simulink model "rp5p1"  (Simulink 10.1)
settings: Solver=ode5  StartTime=0.0  StopTime=10  FixedStep=0.001  RelTol=1e-3
libraries: simulink x3, Solver_SF x1
settings Model: Creator=lancer  LastModifiedBy=Administrator
settings DataIOCC: SaveFormat=Dataset
settings OptimizationCC: LifeSpan=auto
settings DebuggingCC: UnderspecifiedInitializationDetection=Simplified  MergeDetectMultiDrivingBlocksExec=error  SFUnexpectedBacktrackingDiag=error  SFNoUnconditionalDefaultTransitionDiag=error  SFExecutionAtInitializationDiag=warning
settings HardwareCC: ProdBitPerPointer=64  ProdBitPerSizeT=64  ProdBitPerPtrDiffT=64  ProdLargestAtomicFloat=Float  ProdIntDivRoundTo=Zero  ProdEndianess=LittleEndian  ProdWordSize=64  ProdHWDeviceType=Intel->x86-64 (Windows64)
settings ModelReferenceCC: PropagateSignalLabelsOutOfModel=on
settings CodeAppCC: StateflowObjectComments=off
settings GRTTargetCC: TargetLangStandard=C99 (ISO)  CombineOutputUpdateFcns=on  GRTInterface=off
settings ConfigComp: CovMetricSettings=dwe  CovHtmlReporting=off  CovSaveCumulativeToWorkspaceVar=off  CovSaveSingleToWorkspaceVar=off  CovExternalEMLEnable=on

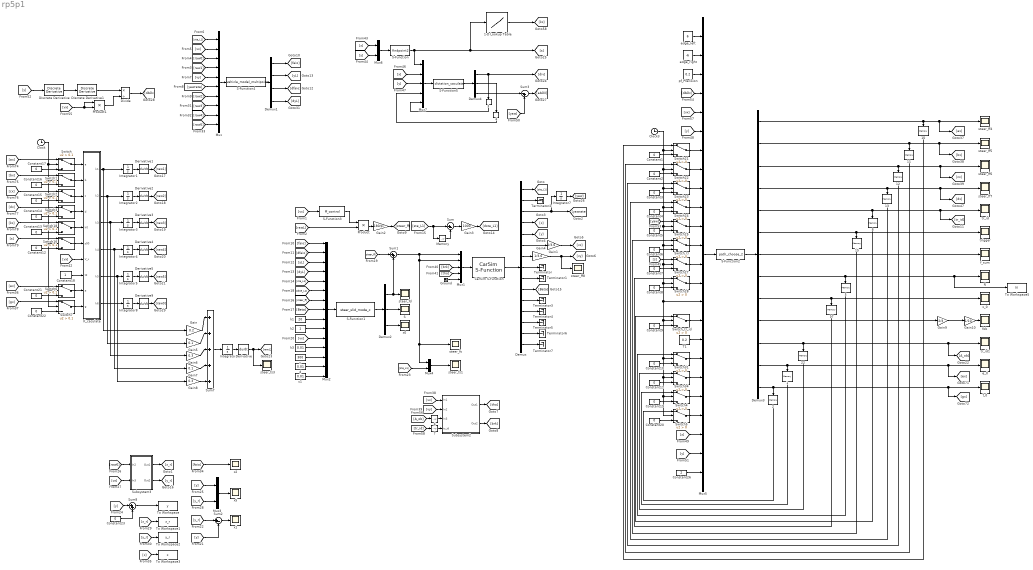
== system rp5p1 ==
  {1..8,10..13,15,17,22} (15 alike) : Memory
  1-D Lookup Table : Lookup_n-D  NumberOfTableDimensions=1  BreakpointsForDimension1=xlsread('cos_road','sheet2','C2:C4002')  Table=xlsread('cos_road','sheet2','F2:F4002')  InternalRulePriority=Speed  RndMeth=Simplest  InputSameDT=on
  CarSim S-Function : Solver_SF/CarSim S-Function  Priority=1  VehicleCode=i_i  SIMFILE=simfile.sim
  Clock : Clock
  Clock3 : Clock
  Constant{1..17,19..23} (22 alike) : Constant  Value=0
  Constant18 : Constant
  Constant26 : Constant  Value=2
  Demux : Demux  Outputs=15
  Demux1 : Demux
  Demux2 : Demux  Outputs=3
  Demux3 : Demux  Outputs=13
  Demux4 : Demux  Outputs=3
  Derivative{,1..5,9} (7 alike) : Derivative
  Discrete Derivative : simulink/Discrete/Discrete Derivative  gainval=1.0  ICPrevScaledInput=0.0  OutMin=[]  OutMax=[]  OutDataType=fixdt(1, 16)  OutScaling=2^-10  DoSatur=off
  Discrete Derivative1 : simulink/Discrete/Discrete Derivative  gainval=1.0  ICPrevScaledInput=0.0  OutMin=[]  OutMax=[]  OutDataType=fixdt(1, 16)  OutScaling=2^-10  DoSatur=off
  Divide : Product  Inputs=*/
  Gain : Gain  Gain=0.2
  Gain1 : Gain  Gain=1/3.6
  Gain10 : Gain  Gain=1/10
  Gain2 : Gain  Gain=180/pi
  Gain3 : Gain  Gain=1000
  Gain4 : Gain  Gain=1/3.6
  Gain5 : Gain  Gain=0.1
  Gain6 : Gain  Gain=0.3
  Gain7 : Gain  Gain=0.1
  Gain8 : Gain  Gain=0.3
  Gain9 : Gain  Gain=2/3
  Ground : Ground
  Integrator{,1..5,7..8} (8 alike) : Integrator
  K_caculate : Subsystem
  Memory : Memory
  Mux : Mux  Inputs=10
  Mux1 : Mux  Inputs=5
  Mux2 : Mux  Inputs=15
  Mux3 : Mux  Inputs=2
  Mux4 : Mux  Inputs=2
  Mux5 : Mux  Inputs=24
  Mux6 : Mux  Inputs=2
  Mux7 : Mux  Inputs=5
  N : Scope
  Product : Product
  Product1 : Product
  S : Scope
  S-Function : S-Function  FunctionName=findpoint2  Parameters=path_data_2  SFunctionDeploymentMode=off  EnableBusSupport=off
  S-Function1 : S-Function  FunctionName=steer_slid_mode_c  SFunctionDeploymentMode=off  EnableBusSupport=off
  S-Function2 : S-Function  FunctionName=path_choose_2  Parameters=path_data_2  SFunctionDeploymentMode=off  EnableBusSupport=off
  S-Function3 : S-Function  FunctionName=ff_control  SFunctionDeploymentMode=off  EnableBusSupport=off
  S-Function4 : S-Function  FunctionName=vehicle_model_multipoint  SFunctionDeploymentMode=off  EnableBusSupport=off
  S-Function5 : S-Function  FunctionName=diviation_caculate  Parameters=path_data_2  SFunctionDeploymentMode=off  EnableBusSupport=off
  Subsystem2 : Subsystem
  Subsystem3 : Subsystem
  Sum : Sum  Inputs=|+-
  Sum1 : Sum  Inputs=|++
  Sum2 : Sum  Inputs=|+-
  Sum3 : Sum  Inputs=|-+
  Sum7 : Sum  Inputs=|+++++
  Sum8 : Sum  Inputs=|++
  Switch{,1..3,6..7,16,18} (8 alike) : Switch  Criteria=u2 > Threshold  Threshold=0.1
  Switch{4..5,21..25,27..28,31,34} (11 alike) : Switch  Criteria=u2 > Threshold
  Switch_tr : Switch  Criteria=u2 > Threshold
  Switch_tr_id : Switch  Criteria=u2 > Threshold
  T1 : Constant  Value=0.2
  Terminator{,1..7} (8 alike) : Terminator
  To Workspace : ToWorkspace  VariableName=y  SaveFormat=Timeseries  SampleTime=-1
  To Workspace1 : ToWorkspace  VariableName=x_r  SaveFormat=Timeseries  SampleTime=-1
  To Workspace2 : ToWorkspace  VariableName=y_r  SaveFormat=Timeseries  SampleTime=-1
  To Workspace3 : ToWorkspace  VariableName=x  SaveFormat=Timeseries  SampleTime=-1
  To Workspace5 : ToWorkspace  VariableName=N  SaveFormat=Timeseries  SampleTime=-1
  c : Constant  Value=300
  c1 : Constant  Value=0.01
  d : Constant  Value=0.01
  e_0 : Scope
  edge_left : Constant  Value=6
  edge_right : Constant  Value=-6
  f_0 : Scope
  f_sum : Scope
  fob : Scope
  k1 : Constant  Value=20
  k2 : Constant
  k3 : Constant  Value=0.01
  pf_Precision : Constant  Value=0.2
  steer_fd : Scope
  steer_ff{4..8} (5 alike) : Scope
  steer_fs : Scope
  steer_fs1 : Scope
  steer_fs3 : Scope
  tr_id : Scope
  tr_id1 : Scope
  trigger : Scope
  x{0..2,5} (4 alike) : Scope
  x_0 : Scope
  wires:
  Demux/1 -> [ste_L1]
  Demux/2 -> Terminator2/1
  Demux/4 -> [x]
  Demux/5 -> [y]
  Demux/8 -> Terminator/1
  Demux/9 -> Terminator1/1
  Demux/10 -> [Beta]
  Demux/11 -> Terminator3/1
  Demux/12 -> Terminator4/1
  Demux/13 -> Terminator5/1
  Demux/14 -> Terminator6/1
  [vx] -> S-Function3/1
  S-Function3/1 -> Product/1
  [rawL] -> Product/2
  Mux/1 -> S-Function4/1
  [raw1] -> Mux/4
  [raw0] -> Mux/3
  [vx] -> Mux/2
  [ste_L1] -> Mux/1
  [vy] -> Mux/5
  [yawrate] -> Mux/6
  S-Function4/1 -> Demux1/1
  Mux2/1 -> S-Function1/1
  [faio] -> Mux2/1
  [dfaio] -> Mux2/2
  [yL] -> Mux2/3
  [dyL] -> Mux2/4
  [ste_L1] -> Mux2/5
  [dste_L1] -> Mux2/6
  [steer_ff] -> Mux2/7
  [Beta] -> Mux2/8
  k1/1 -> Mux2/9
  k2/1 -> Mux2/10
  [vx] -> Mux2/11
  k3/1 -> Mux2/12
  c/1 -> Mux2/13
  d/1 -> Mux2/14
  c1/1 -> Mux2/15
  [ste_L1] -> Memory/1, Sum/1
  Memory/1 -> Sum/2
  S-Function1/1 -> Demux2/1
  Product/1 -> Gain2/1
  Gain2/1 -> [steer_ff]
  [steer_ff] -> Sum1/1
  Demux2/1 -> steer_fd/1, Sum1/2
  Sum1/1 -> Mux4/1, steer_fs/1, Mux1/2, Mux1/1
  Demux2/2 -> S/1
  Demux2/3 -> x0/1
  Sum/1 -> Gain3/1
  Gain3/1 -> [dste_L1]
  Demux/6 -> Gain1/1
  Gain1/1 -> [vx]
  Gain4/1 -> steer_ff8/1, [vy]
  Demux/7 -> Gain4/1
  [raw0] -> Subsystem3/1(In2)
  [vx] -> Subsystem3/2(In3)
  Subsystem3/1(Out1) -> [x_r]
  Subsystem3/2(Out2) -> [y_r]
  [y_r] -> Sum2/1
  [y] -> Sum2/2
  [y] -> Mux3/1
  [y_r] -> Mux3/2
  Mux3/1 -> x5/1
  Sum2/1 -> x1/1
  [ste_L1] -> Mux4/2
  Mux4/1 -> steer_fs1/1
  [x_r] -> To Workspace1/1
  [y_r] -> To Workspace2/1
  [raw2] -> Mux/7
  [raw3] -> Mux/8
  [raw4] -> Mux/9
  [raw5] -> Mux/10
  [faio] -> x2/1
  Mux1/1 -> CarSim S-Function/1
  CarSim S-Function/1 -> Demux/1
  [x] -> To Workspace3/1
  [brk] -> Mux1/3
  [tho] -> Mux1/4
  Demux1/1 -> [faio]
  Demux1/3 -> [dfaio]
  Subsystem2/2(Out2) -> [brk]
  [vx] -> Subsystem2/1(In1)
  Subsystem2/1(Out1) -> [tho]
  [vy] -> Subsystem2/2(In2)
  Mux5/1 -> S-Function2/1
  Demux3/13 -> 2/1, [gx], f_0/1
  Demux3/12 -> 1/1, e_0/1, [ex]
  Constant8/1 -> Switch28/3
  17/1 -> Switch28/1
  Constant10/1 -> Switch31/3
  Constant9/1 -> Switch_tr_id/3
  Constant2/1 -> Switch22/3
  Demux3/2 -> steer_ff5/1, [bx], 11/1
  12/1 -> Switch23/1
  Demux3/4 -> steer_ff7/1, [dx], 13/1
  Constant11/1 -> Switch34/3
  10/1 -> Switch21/1
  Demux3/1 -> steer_ff4/1, [ax], 10/1
  13/1 -> Switch24/1
  15/1 -> Switch_tr/1
  11/1 -> Switch22/1
  Constant1/1 -> Switch21/3
  Demux3/3 -> steer_ff6/1, [cx], 12/1
  Constant4/1 -> Switch24/3
  Constant7/1 -> Switch27/3
  Constant3/1 -> Switch23/3
  S-Function2/1 -> Demux3/1
  Demux3/7 -> f_sum/1
  Constant6/1 -> Switch_tr/3
  22/1 -> Switch34/1
  Demux3/6 -> trigger/1, 15/1
  Constant5/1 -> Switch25/3
  Demux3/11 -> [A_ob], tr_id1/1, 22/1
  Demux3/9 -> 17/1, x_0/1
  Switch34/1 -> Mux5/19
  Switch31/1 -> Mux5/18
  Switch_tr_id/1 -> Mux5/16
  T1/1 -> Mux5/17
  [dAGx] -> Mux5/4
  [vx] -> Mux5/5
  [y] -> Mux5/6
  Switch21/1 -> Mux5/7
  Switch22/1 -> Mux5/8
  Switch23/1 -> Mux5/9
  Switch24/1 -> Mux5/10
  Switch25/1 -> Mux5/11
  Switch_tr/1 -> Mux5/12
  Switch28/1 -> Mux5/14
  Switch27/1 -> Mux5/13
  edge_left/1 -> Mux5/1
  edge_right/1 -> Mux5/2
  pf_Precision/1 -> Mux5/3
  K_caculate/4(k4) -> Gain7/1, Integrator4/1
  K_caculate/2(k2) -> Gain5/1, Integrator2/1
  Switch2/1 -> K_caculate/3(c)
  Constant18/1 -> K_caculate/8(t2)
  K_caculate/3(k3) -> Gain6/1, Integrator3/1
  [kx] -> Switch18/1
  Switch1/1 -> K_caculate/2(b)
  [vx] -> K_caculate/7(V_x)
  Constant17/1 -> Switch/3
  Switch/1 -> K_caculate/1(a)
  Switch3/1 -> K_caculate/4(d)
  K_caculate/5(k5) -> Gain8/1, Integrator5/1
  [ax] -> Switch/1
  Switch18/1 -> K_caculate/5(k0)
  [cx] -> Switch2/1
  [s] -> Switch16/1
  Constant13/1 -> Switch18/3
  [bx] -> Switch1/1
  Constant14/1 -> Switch3/3
  [dx] -> Switch3/1
  Constant15/1 -> Switch2/3
  Constant12/1 -> Switch16/3
  Switch16/1 -> K_caculate/6(s00)
  Constant16/1 -> Switch1/3
  Gain/1 -> Sum7/1
  Gain8/1 -> Sum7/5
  Gain7/1 -> Sum7/4
  Gain6/1 -> Sum7/3
  Gain5/1 -> Sum7/2
  Integrator/1 -> Derivative/1
  Sum7/1 -> Integrator/1
  Derivative/1 -> [rawL], steer_fs3/1
  Integrator1/1 -> Derivative1/1
  Derivative1/1 -> [raw1]
  Integrator2/1 -> Derivative2/1
  Derivative2/1 -> [raw2]
  Integrator3/1 -> Derivative3/1
  Integrator4/1 -> Derivative4/1
  Integrator5/1 -> Derivative5/1
  Derivative4/1 -> [raw4]
  Derivative5/1 -> [raw5]
  Derivative3/1 -> [raw3]
  [y] -> Sum8/1
  Sum8/1 -> To Workspace/1
  Constant19/1 -> Switch4/3
  Constant20/1 -> Switch5/3
  Clock3/1 -> Switch5/2, Switch4/2, Switch34/2, Switch31/2, Switch_tr_id/2, Mux5/15, Switch28/2, Switch27/2, Switch_tr/2, Switch25/2, Switch24/2, Switch23/2, Switch22/2, Switch21/2
  Switch5/1 -> Mux5/21
  1/1 -> Switch4/1
  2/1 -> Switch5/1
  [ex] -> Switch6/1
  Constant21/1 -> Switch6/3
  Switch6/1 -> K_caculate/9(e)
  Clock/1 -> Switch7/2, Switch6/2, Switch16/2, Switch18/2, Switch3/2, Switch2/2, Switch1/2, Switch/2
  [gx] -> Switch7/1
  Constant22/1 -> Switch7/3
  Switch7/1 -> K_caculate/10(g)
  Mux6/1 -> S-Function/1
  [x] -> Mux6/1
  [y] -> Mux6/2
  S-Function/1 -> 1-D Lookup Table/1, [s], Mux7/1
  [s] -> Switch27/1
  Constant23/1 -> Sum8/2
  Mux7/1 -> S-Function5/1
  [x] -> Mux7/2
  [y] -> Mux7/3
  S-Function5/1 -> Demux4/1
  Demux4/2 -> 4/1
  3/1 -> Mux7/5
  4/1 -> Mux7/4
  1-D Lookup Table/1 -> [kx]
  Demux3/8 -> 5/1, To Workspace5/1, N/1
  Integrator7/1 -> [yaw]
  Switch4/1 -> Mux5/20
  Demux4/3 -> Sum3/1
  Demux3/5 -> 8/1, tr_id/1, [tr_id]
  [yaw] -> Switch25/1
  Demux4/1 -> [div], 3/1
  [yaw] -> Sum3/2
  [x] -> Mux5/22
  [y] -> Mux5/23
  Constant26/1 -> Mux5/24
  Discrete Derivative/1 -> Discrete Derivative1/1
  Derivative9/1 -> [raw0]
  Integrator8/1 -> Derivative9/1
  K_caculate/1(k1) -> Gain/1, Integrator1/1
  K_caculate/6(k6) -> Integrator8/1
  Demux1/4 -> [dyL]
  Demux1/2 -> [yL]
  [y] -> Discrete Derivative/1
  Demux/3 -> Integrator7/1, [yawrate]
  Demux/15 -> Terminator7/1
  Ground/1 -> Mux1/5
  Divide/1 -> [dAGx]
  Discrete Derivative1/1 -> Divide/1
  [vx] -> Product1/2, Product1/1
  Product1/1 -> Divide/2
  [A_ob] -> 6/1
  6/1 -> Subsystem2/3(In3)
  [tr_id] -> 7/1
  7/1 -> Subsystem2/4(tr_id)
  8/1 -> Switch_tr_id/1
  5/1 -> Switch31/1
  Demux3/10 -> Gain9/1
  Gain9/1 -> Gain10/1
  Gain10/1 -> fob/1
  Sum3/1 -> [aAGX]

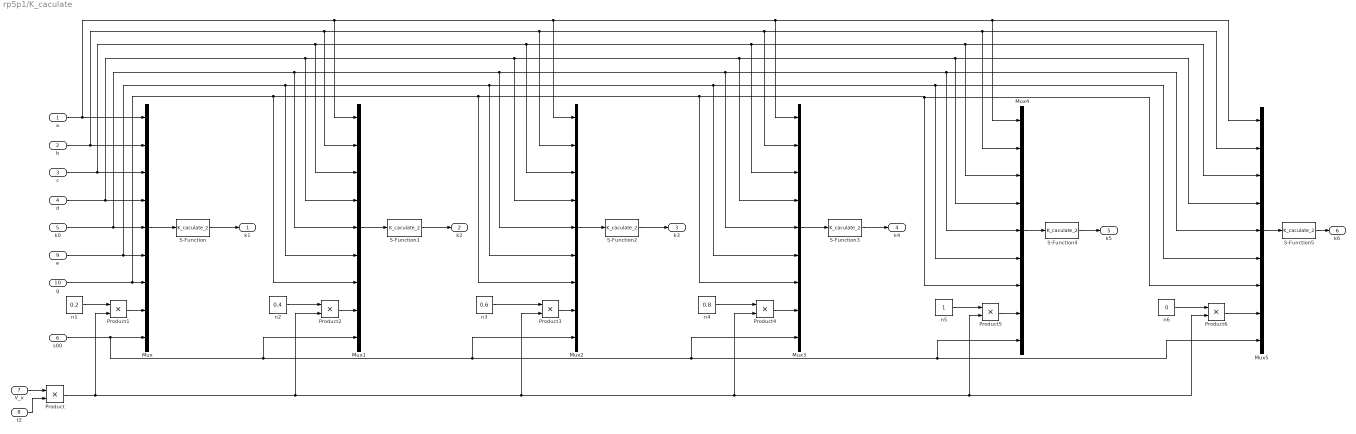
== system rp5p1/K_caculate ==
  a : Inport
  b : Inport  Port=2
  c : Inport  Port=3
  d : Inport  Port=4
  k0 : Inport  Port=5
  s00 : Inport  Port=6
  V_x : Inport  Port=7
  t2 : Inport  Port=8
  e : Inport  Port=9
  g : Inport  Port=10
  Mux{,1..5} (6 alike) : Mux  Inputs=9
  Product{,1..6} (7 alike) : Product
  S-Function{,1..5} (6 alike) : S-Function  FunctionName=K_caculate_2  SFunctionDeploymentMode=off  EnableBusSupport=off
  n1 : Constant  Value=0.2
  n2 : Constant  Value=0.4
  n3 : Constant  Value=0.6
  n4 : Constant  Value=0.8
  n5 : Constant
  n6 : Constant  Value=0
  k1 : Outport  VectorParamsAs1DForOutWhenUnconnected=off
  k2 : Outport  Port=2  VectorParamsAs1DForOutWhenUnconnected=off
  k3 : Outport  Port=3  VectorParamsAs1DForOutWhenUnconnected=off
  k4 : Outport  Port=4  VectorParamsAs1DForOutWhenUnconnected=off
  k5 : Outport  Port=5  VectorParamsAs1DForOutWhenUnconnected=off
  k6 : Outport  Port=6  VectorParamsAs1DForOutWhenUnconnected=off
  wires:
  s00/1 -> Mux/9, Mux1/9, Mux2/9, Mux5/9, Mux4/9, Mux3/9
  Mux/1 -> S-Function/1
  S-Function/1 -> k1/1
  k0/1 -> Mux1/5, Mux2/5, Mux3/5, Mux5/5, Mux4/5, Mux/5
  a/1 -> Mux/1, Mux1/1, Mux2/1, Mux3/1, Mux5/1, Mux4/1
  c/1 -> Mux1/3, Mux2/3, Mux3/3, Mux4/3, Mux5/3, Mux/3
  d/1 -> Mux1/4, Mux2/4, Mux3/4, Mux5/4, Mux4/4, Mux/4
  Mux1/1 -> S-Function1/1
  S-Function1/1 -> k2/1
  Mux2/1 -> S-Function2/1
  S-Function2/1 -> k3/1
  Mux3/1 -> S-Function3/1
  S-Function3/1 -> k4/1
  Mux4/1 -> S-Function4/1
  S-Function4/1 -> k5/1
  b/1 -> Mux/2, Mux1/2, Mux2/2, Mux3/2, Mux4/2, Mux5/2
  V_x/1 -> Product/1
  t2/1 -> Product/2
  n1/1 -> Product1/1
  n2/1 -> Product2/1
  n3/1 -> Product3/1
  n4/1 -> Product4/1
  n5/1 -> Product5/1
  e/1 -> Mux1/6, Mux2/6, Mux3/6, Mux5/6, Mux4/6, Mux/6
  g/1 -> Mux1/7, Mux2/7, Mux3/7, Mux5/7, Mux4/7, Mux/7
  Product1/1 -> Mux/8
  Product5/1 -> Mux4/8
  Product4/1 -> Mux3/8
  Product3/1 -> Mux2/8
  Product2/1 -> Mux1/8
  S-Function5/1 -> k6/1
  Mux5/1 -> S-Function5/1
  n6/1 -> Product6/1
  Product6/1 -> Mux5/8
  Product/1 -> Product3/2, Product6/2, Product5/2, Product4/2, Product2/2, Product1/2

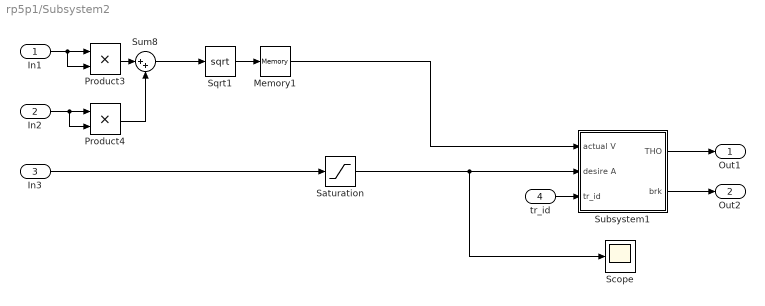
== system rp5p1/Subsystem2 ==
  In1 : Inport
  In2 : Inport  Port=2
  In3 : Inport  Port=3
  tr_id : Inport  Port=4
  Memory1 : Memory
  Product3 : Product
  Product4 : Product
  Saturation : Saturate  UpperLimit=5  LowerLimit=-5
  Scope : Scope
  Sqrt1 : Sqrt  SaturateOnIntegerOverflow=on
  Subsystem1 : Subsystem
  Sum8 : Sum  Inputs=|++
  Out1 : Outport  VectorParamsAs1DForOutWhenUnconnected=off
  Out2 : Outport  Port=2  VectorParamsAs1DForOutWhenUnconnected=off
  wires:
  Subsystem1/1(THO) -> Out1/1
  Sqrt1/1 -> Memory1/1
  Sum8/1 -> Sqrt1/1
  Subsystem1/2(brk) -> Out2/1
  In2/1 -> Product4/2, Product4/1
  Product4/1 -> Sum8/2
  Product3/1 -> Sum8/1
  In1/1 -> Product3/2, Product3/1
  Memory1/1 -> Subsystem1/1(actual V)
  Saturation/1 -> Subsystem1/2(desire A), Scope/1
  In3/1 -> Saturation/1
  tr_id/1 -> Subsystem1/3(tr_id)

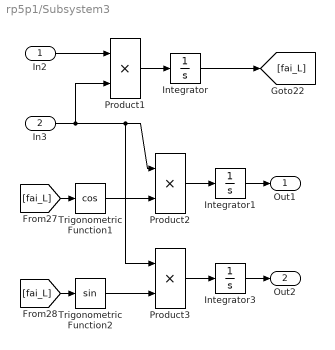
== system rp5p1/Subsystem3 ==
  In2 : Inport
  In3 : Inport  Port=2
  Integrator : Integrator
  Integrator1 : Integrator
  Integrator3 : Integrator
  Product1 : Product  RndMeth=Zero
  Product2 : Product  RndMeth=Zero
  Product3 : Product  RndMeth=Zero
  Trigonometric Function1 : Trigonometry  Operator=cos
  Trigonometric Function2 : Trigonometry
  Out1 : Outport  VectorParamsAs1DForOutWhenUnconnected=off
  Out2 : Outport  Port=2  VectorParamsAs1DForOutWhenUnconnected=off
  wires:
  In3/1 -> Product1/2, Product3/1, Product2/1
  Product1/1 -> Integrator/1
  [fai_L] -> Trigonometric Function1/1
  Trigonometric Function1/1 -> Product2/2
  Product2/1 -> Integrator1/1
  [fai_L] -> Trigonometric Function2/1
  Trigonometric Function2/1 -> Product3/2
  Product3/1 -> Integrator3/1
  Integrator/1 -> [fai_L]
  In2/1 -> Product1/1
  Integrator1/1 -> Out1/1
  Integrator3/1 -> Out2/1

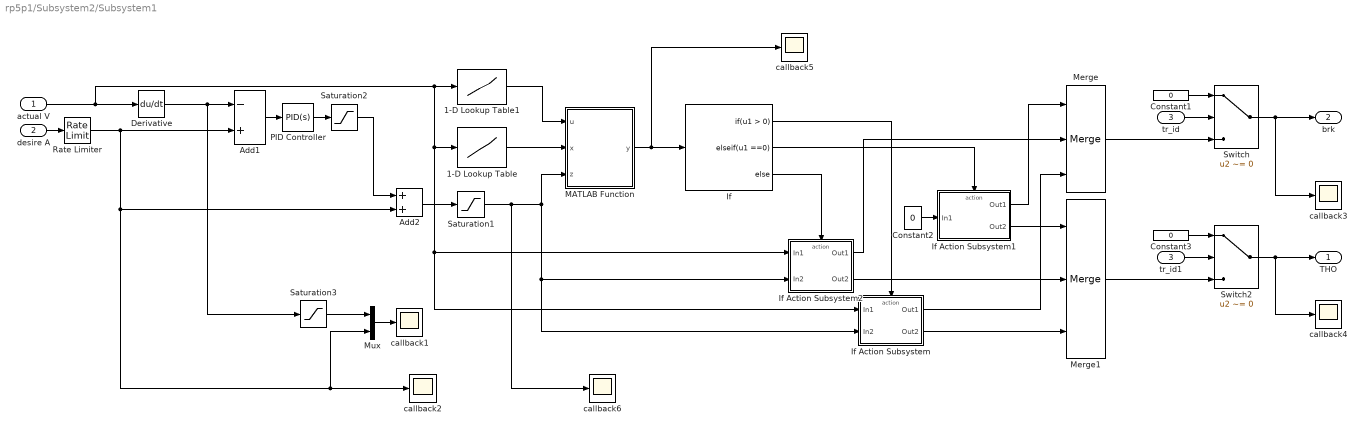
== system rp5p1/Subsystem2/Subsystem1 ==
  actual V : Inport
  desire A : Inport  Port=2
  tr_id : Inport  Port=3
  1-D Lookup Table : Lookup_n-D  NumberOfTableDimensions=1  BreakpointsForDimension1=xlsread('tho0brk0','sheet4','A2:A16')  Table=xlsread('tho0brk0','sheet4','B2:B16')  InternalRulePriority=Speed  RndMeth=Simplest  InputSameDT=on
  1-D Lookup Table1 : Lookup_n-D  NumberOfTableDimensions=1  BreakpointsForDimension1=xlsread('tho0brk0','sheet3','A2:A29')  Table=xlsread('tho0brk0','sheet3','B2:B29')  InternalRulePriority=Speed  RndMeth=Simplest  InputSameDT=on
  Add1 : Sum  Inputs=-+
  Add2 : Sum
  Constant1 : Constant  Value=0
  Constant2 : Constant  Value=0
  Constant3 : Constant  Value=0
  Derivative : Derivative
  If : If  ElseIfExpressions=u1 ==0
  If Action Subsystem : Subsystem  TreatAsAtomicUnit=on
  If Action Subsystem1 : Subsystem  TreatAsAtomicUnit=on
  If Action Subsystem2 : Subsystem  TreatAsAtomicUnit=on
  MATLAB Function : MATLAB Function  TreatAsAtomicUnit=on
  Merge : Merge  Inputs=3
  Merge1 : Merge  Inputs=3
  Mux : Mux  Inputs=2
  PID Controller : simulink/Continuous/PID Controller  Controller=PID  Form=Parallel  TimeDomain=Continuous-time  UseExternalTs=off  SampleTime=-1  IntegratorMethod=Forward Euler  FilterMethod=Forward Euler  ControllerParametersSource=internal  P=5  I=0.01  D=0.005  UseFilter=on  N=100  TunerSelectOption=Transfer Function Based (PID Tuner App)  InitialConditionSource=internal  InitialConditionForIntegrator=0  InitialConditionForFilter=0  DifferentiatorICPrevScaledInput=0  ExternalReset=none  TrackingMode=off  Kt=1  LimitOutput=off  UpperSaturationLimit=inf  LowerSaturationLimit=-inf  LinearizeAsGain=on  AntiWindupMode=none  Kb=1  POutMin=[]  POutMax=[]  IOutMin=[]  IOutMax=[]  DOutMin=[]  DOutMax=[]  NOutMin=[]  NOutMax=[]  SumOutMin=[]  SumOutMax=[]  SaturationOutMin=[]  SaturationOutMax=[]  PParamMin=[]  PParamMax=[]  IParamMin=[]  IParamMax=[]  DParamMin=[]  DParamMax=[]  NParamMin=[]  NParamMax=[]  KbParamMin=[]  KbParamMax=[]  KtParamMin=[]  KtParamMax=[]  KbOutMin=[]  KbOutMax=[]  KtOutMin=[]  KtOutMax=[]  IntegratorOutMin=[]  IntegratorOutMax=[]  FilterOutMin=[]  FilterOutMax=[]  SumI1OutMin=[]  SumI1OutMax=[]  SumI2OutMin=[]  SumI2OutMax=[]  SumI3OutMin=[]  SumI3OutMax=[]  SumI4OutMin=[]  SumI4OutMax=[]  SumDOutMin=[]  SumDOutMax=[]  DifferentiatorOutMin=[]  DifferentiatorOutMax=[]  FilterDiffOutCoefMin=[]  FilterDiffOutCoefMax=[]  ReciprocalOutMin=[]  ReciprocalOutMax=[]  SumDenOutMin=[]  SumDenOutMax=[]  SumNumOutMin=[]  SumNumOutMax=[]  DivideOutMin=[]  DivideOutMax=[]  UdiffTsProdOutMin=[]  UdiffTsProdOutMax=[]  NTsProdOutMin=[]  NTsProdOutMax=[]  UintegralTsProdOutMin=[]  UintegralTsProdOutMax=[]  UngainTsProdOutMin=[]  UngainTsProdOutMax=[]  IntegratorContinuousStateAttributes=''  IntegratorStateMustResolveToSignalObject=off  IntegratorRTWStateStorageClass=Auto  FilterContinuousStateAttributes=''  FilterStateMustResolveToSignalObject=off  FilterRTWStateStorageClass=Auto  ParallelPVariant=InternalParameters  IdealPVariant=Disabled  IVariant=InternalParameters  DVariant=InternalParameters  IntegratorVariant=Continuous  SatVariant=Disabled  AWVariant=Passthrough  PCopyVariant=Disabled  TRVariant=Disabled  FdbkBlocksVariant=Forward  IdealPFdbkVariant=Disabled  SatFdbkVariant=Disabled  DerivativeFilterVariant=ContFilter  NVariant=InternalParameters  NCopyVariant=Disabled  FilterICVariant=InternalICsFilter  IntegratorICVariant=InternalICs  ExternalResetVariant=Disabled  TRSumVariant=Passthrough  SumFdbkVariant=Disabled  SumVariant=Sum_PID  TsampFilterVariant=InternalTs  TsampNgainVariant=Passthrough  TsampIntegralVariant=Passthrough
  Rate Limiter : RateLimiter  RisingSlewLimit=5  FallingSlewLimit=-5  SampleTimeMode=inherited
  Saturation1 : Saturate  UpperLimit=5.4  LowerLimit=-5
  Saturation2 : Saturate  UpperLimit=5.4  LowerLimit=-5
  Saturation3 : Saturate  UpperLimit=5.4  LowerLimit=-5
  Switch : Switch  Criteria=u2 ~= 0
  Switch2 : Switch  Criteria=u2 ~= 0
  callback{1..6} (6 alike) : Scope
  tr_id1 : InportShadow  Port=3
  THO : Outport  VectorParamsAs1DForOutWhenUnconnected=off
  brk : Outport  Port=2  VectorParamsAs1DForOutWhenUnconnected=off
  wires:
  If Action Subsystem2/1(Out1) -> Merge/2
  Saturation1/1 -> callback6/1, If Action Subsystem/2(In2), If Action Subsystem2/2(In2), MATLAB Function/3(z)
  If Action Subsystem/2(Out2) -> Merge1/3
  If Action Subsystem1/1(Out1) -> Merge/1
  If/2 -> If Action Subsystem1/Action
  Add1/1 -> PID Controller/1
  If/1 -> If Action Subsystem/Action
  If Action Subsystem/1(Out1) -> Merge/3
  If/3 -> If Action Subsystem2/Action
  Add2/1 -> Saturation1/1
  Rate Limiter/1 -> Add1/2, Add2/2, Mux/2, callback2/1
  Constant2/1 -> If Action Subsystem1/1(In1)
  If Action Subsystem2/2(Out2) -> Merge1/2
  1-D Lookup Table/1 -> MATLAB Function/2(x)
  If Action Subsystem1/2(Out2) -> Merge1/1
  Saturation2/1 -> Add2/1
  1-D Lookup Table1/1 -> MATLAB Function/1(u)
  MATLAB Function/1(y) -> callback5/1, If/1
  actual V/1 -> 1-D Lookup Table/1, If Action Subsystem2/1(In1), If Action Subsystem/1(In1), 1-D Lookup Table1/1, Derivative/1
  desire A/1 -> Rate Limiter/1
  PID Controller/1 -> Saturation2/1
  Switch/1 -> callback3/1, brk/1
  Switch2/1 -> THO/1, callback4/1
  Constant3/1 -> Switch2/1
  tr_id/1 -> Switch/2
  tr_id1/1 -> Switch2/2
  Merge/1 -> Switch/3
  Constant1/1 -> Switch/1
  Merge1/1 -> Switch2/3
  Derivative/1 -> Saturation3/1, Add1/1
  Mux/1 -> callback1/1
  Saturation3/1 -> Mux/1

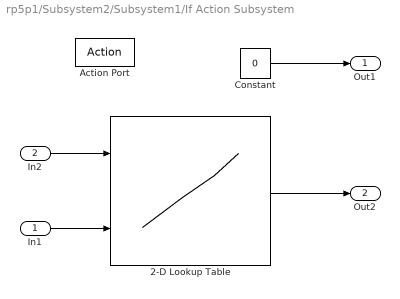
== system rp5p1/Subsystem2/Subsystem1/If Action Subsystem ==
  In1 : Inport
  In2 : Inport  Port=2
  Action Port : ActionPort  ActionPortLabel=if { }
  2-D Lookup Table : Lookup_n-D  BreakpointsForDimension1=xlsread('tho-v-a','sheet4','A3:A38')  BreakpointsForDimension2=xlsread('tho-v-a','sheet4','B2:P2')  Table=xlsread('tho-v-a','sheet4','B3:P38')  InternalRulePriority=Speed  RndMeth=Simplest  InputSameDT=on
  Constant : Constant  Value=0
  Out1 : Outport  VectorParamsAs1DForOutWhenUnconnected=off
  Out2 : Outport  Port=2  VectorParamsAs1DForOutWhenUnconnected=off
  wires:
  Constant/1 -> Out1/1
  2-D Lookup Table/1 -> Out2/1
  In2/1 -> 2-D Lookup Table/1
  In1/1 -> 2-D Lookup Table/2

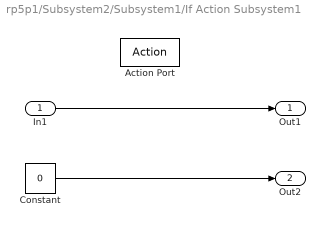
== system rp5p1/Subsystem2/Subsystem1/If Action Subsystem1 ==
  In1 : Inport
  Action Port : ActionPort  ActionPortLabel=elseif { }
  Constant : Constant  Value=0
  Out1 : Outport  VectorParamsAs1DForOutWhenUnconnected=off
  Out2 : Outport  Port=2  VectorParamsAs1DForOutWhenUnconnected=off
  wires:
  In1/1 -> Out1/1
  Constant/1 -> Out2/1

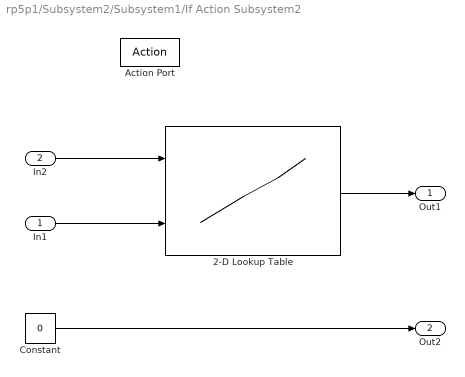
== system rp5p1/Subsystem2/Subsystem1/If Action Subsystem2 ==
  In1 : Inport
  In2 : Inport  Port=2
  Action Port : ActionPort  ActionPortLabel=else { }
  2-D Lookup Table : Lookup_n-D  BreakpointsForDimension1=xlsread('brk-v-a','sheet3','A3:A28')  BreakpointsForDimension2=xlsread('brk-v-a','sheet3','B2:P2')  Table=xlsread('brk-v-a','sheet3','B3:P28')  InternalRulePriority=Speed  RndMeth=Simplest  InputSameDT=on
  Constant : Constant  Value=0
  Out1 : Outport  VectorParamsAs1DForOutWhenUnconnected=off
  Out2 : Outport  Port=2  VectorParamsAs1DForOutWhenUnconnected=off
  wires:
  2-D Lookup Table/1 -> Out1/1
  Constant/1 -> Out2/1
  In2/1 -> 2-D Lookup Table/1
  In1/1 -> 2-D Lookup Table/2

== matlab function Subsystem2/Subsystem1/MATLAB Function ==
  data: u input double; y output double; x input double; z input double
function y = fcn(u, x, z)
if z>u
    y=1;
elseif z<u&&z>x
    y=0;
elseif z<x
    y=-1;
else
    y=5;
end
